simulink model "Electrical_System_2018b_obfs"  (R2019b)
settings: Solver=VariableStepAuto  StartTime=0.0  StopTime=5  RelTol=1e-3  AbsTol=1e-3  EnableMultiTasking=on
InitFcn:
  | Steady_State_Initialisation;
StopFcn:
  | %sscexplore(simlog);
  | %Logging
undefined symbols (not defined in the file): abrlhklxvp, aexgmhuedq, afmfmjnutg, afpphrjpnc, ahuxbyvruc, alarvljztt, amxnyqmnuw, aodrlwvqie, aolhmuplyq, aqpmguuqkg, auesgwirzl, aurophlnng, awamelrhru, ayfhvxflxn, azxkacuhqc, babszerikg, bawhdqanwq, bevoqecvei, bltjvqbchx, bmqsuewujl, bsmyqjfgnf, btvjbsmnve, bywgxqeadw, bziaduxaer, bzmcmdqocb, bzsvyvetat, ccsjnrbsih, cdvenygxwh, cedkrnslhx, cjheorclzs, cjrdshrtqx, ckhavyhcza, ckxewznhlz, cmrcgyiplk, conenicnws, cqkejbgjnn, csfnuwymhe, cunupkhwbh, cwzfvzuxxh, dcadmadufn, dcfponivnv, ddtrqjrhjn, dfhoxvkqas, dfrhtcwpne, dfvomcagjv, djijwylxea, dnmeqksrrm, dnzewbdkaa, dsqcykyxav, dtswwlttmm, ecumpidjtv, edegaywrct, ejjjsmnejc, eknqnehjdz, emvdetzouf, esxbqkbahr, etnkkbreiq, eunoiiiirw, ewewcuedir, fatkfxdhtc ... (+386)
libraries: fl_lib x802, ee_lib x362, fl_ps_legacy_lib x160, nesl_utility x85
(part 13 of 26)

== system Electrical_System_2018b_obfs/Redacted_1221/Redacted_7996/Redacted_1/Redacted_4377/Redacted_6082/Redacted_7871 ==
  Redacted_1150 : ee_lib/Passive/Thermal/Thermal Resistor  R=wnyhcrensu K/W  T_specify=off  T_priority=None  T=hfmwboisgl K  T_nominal_specify=off  T_nominal_unit=K  T_nominal_value=omfgbcxeiw  Q_specify=off  Q_priority=None  Q=jyeccfnuuv W  Q_nominal_specify=off  Q_nominal_unit=W  Q_nominal_value=kbomgljmud
      settings: SourceProductName=Simscape Electrical  SourceProductBaseCode=PS  InternalSimscapePortConfiguration="{\"Bottom\":[],\"Left\":[{\"id\":\"A\",\"label\":\"A\",\"type\":\"foundation.thermal.thermal\"}],\"Right\":[{\"id\":\"B\",\"label\":\"B\",\"type\":\"foundation.thermal.thermal\"}],\"Top\":[]}"
  Redacted_163 : fl_lib/Electrical/Electrical Elements/Switch  R_closed=wdukvpamow Ohm  G_open=xulqxrrjnv 1/Ohm  Threshold=qhmovogayg  i_specify=off  i_priority=None  i=uohgsyxugo A  i_nominal_specify=off  i_nominal_unit=A  i_nominal_value=woebaudwry  v_specify=off  v_priority=None  v=vemtymvmmi V  v_nominal_specify=off  v_nominal_unit=V  v_nominal_value=emvbxsbdsz
      settings: SourceProductName=Simscape
  Redacted_4906 : ee_lib/Semiconductors & Converters/Diode  ModelType=lisxnbujfq  Vf=xetfnwixtl V  Ron=kgggytotak Ohm  Goff=dicegnkmns S  prmExp=fsccnkszzi  I12=rkhncbyaxg A  V12=amfquhqfri V  IS=exemtgyddq A  ec=usfpzulpqi  I1=ugfovaezax A  V1=oljxivlmqp V  RS=dazrmfhoxo Ohm  Tmeas=baitckeesm degC  N_series=hfppshhhyr  N_parallel=rjxplrcndp  Rz=fabwipzqjc Ohm  BV=wyrpdjzqjf V  C_param=qgwqtktiiq  CJ=wbrnhtezpt pF  CJ0=phxqhonqpj pF  VJ=eteydoyhly V  Mgrad=glhtwvcvqy  Vvec=hwlxeyydpv V  Cvec=hxporvcfni pF  FC=gjviwqnvyt  Q_param=ncmzgihjzz  iRM=yvoogxejtg A  iF=qnmfqdbeto A  didt=agfovrodto A/us  trr_factor=frcqxuvvia  trr=hbqrwrvnxm ns  Qrr=fdoqfarsjb s*uA  TT=slfzkacqdx ns  tau=alaeanzbod ns  T_param=nuitneutsg  IS_T2=craloeoioz A  I1_T2=wjjsiamplw A  V1_T2=tewsfpvrmq V  Tmeas2=gxtdnafxpo degC  EG_param=wlioyiusag  EG=cpoejbuzyv eV  XTI_param=dddqpnqtzc  XTI=qrfykfwguz  dBVdT=ucurhhzfza V/K  Tdevice=rczcbfyedr degC  i_specify=off  i_priority=None  i=zzdxemwvng A  i_nominal_specify=off  i_nominal_unit=A  i_nominal_value=kfkirmacjn  v_specify=off  v_priority=None  v=uajyhxnboc V  v_nominal_specify=off  v_nominal_unit=V  v_nominal_value=jqepkydgfh  i_capacitor_specify=off  i_capacitor_priority=None  i_capacitor=rrmwbvgmcc A  i_capacitor_nominal_specify=off  i_capacitor_nominal_unit=A  i_capacitor_nominal_value=pjbytllgoo  v_capacitor_specify=off  v_capacitor_priority=None  v_capacitor=pfzlffxyis V  v_capacitor_nominal_specify=off  v_capacitor_nominal_unit=V  v_capacitor_nominal_value=rwblhtqxum  power_dissipated_specify=off  power_dissipated_priority=None  power_dissipated=ezbuvvjzbd W  power_dissipated_nominal_specify=off  power_dissipated_nominal_unit=W  power_dissipated_nominal_value=bhaqvsgfxr  thermal_network_parameterization=kyfbufrfys  Rth=rdswkjtiwa K/W  Rth_Foster=qshnyhfbmq K/W  thermal_mass_parameterization=gvhwjtzboo  thermal_mass=bdoomqzqok J/K  thermal_mass_Foster=anntstrfod J/K  thermal_time_constant=jfrqkttoqa s  thermal_time_constant_Foster=gslnrdmbpc s  thermal_mass_initial_temperatures=ucxtllsqhb degC
      settings: SourceProductName=Simscape Electrical  InternalSimscapePortConfiguration="{\"Bottom\":[],\"Left\":[{\"id\":\"p\",\"label\":\"\",\"type\":\"foundation.electrical.electrical\"},{\"id\":\"H\",\"label\":\"H\",\"type\":\"foundation.thermal.thermal\"}],\"Right\":[{\"id\":\"n\",\"label\":\"\",\"type\":\"foundation.electrical.electrical\"}],\"Top\":[]}"
  Redacted_5585 : fl_lib/Electrical/Electrical Elements/Switch  R_closed=gnrmopaexe Ohm  G_open=orsehmpisd 1/Ohm  Threshold=uztftemjgo  i_specify=off  i_priority=None  i=beydlfyovg A  i_nominal_specify=off  i_nominal_unit=A  i_nominal_value=iaidkfrlwq  v_specify=off  v_priority=None  v=zwfzhspjsy V  v_nominal_specify=off  v_nominal_unit=V  v_nominal_value=hnducacwcv
      settings: SourceProductName=Simscape
  Redacted_6192 : ee_lib/Semiconductors & Converters/Diode  ModelType=ptnynyqzgs  Vf=tkcshdmnfy V  Ron=etdxecgxkr Ohm  Goff=updvlgzhxi S  prmExp=bdmrzzzqpe  I12=sdcvfvczxq A  V12=qxwxvafkrp V  IS=fjehcmaddz A  ec=rcfxzuuzkz  I1=bbqivzbpbn A  V1=jbzephfaei V  RS=jfqjrslbtb Ohm  Tmeas=nmsknhwbdm degC  N_series=upbnprrhsm  N_parallel=gychkiuesj  Rz=ekjrkafpjm Ohm  BV=izllxqqtbw V  C_param=chrhwjdcia  CJ=zewhvymjzh pF  CJ0=xysumvzksz pF  VJ=plgvwexltq V  Mgrad=lfxmdopixh  Vvec=rhhplxfzfv V  Cvec=btxmrjnrpv pF  FC=gllfdejxcp  Q_param=jqpclwrtup  iRM=uzrdiaqfpb A  iF=zfvqwesedg A  didt=zxsbiuiqyg A/us  trr_factor=sbxmtvfbhj  trr=wpldszobql ns  Qrr=rgofeflbzu s*uA  TT=rydmpcnssa ns  tau=bhbpgrjiqy ns  T_param=utvpupdfuz  IS_T2=hbepvkcqcu A  I1_T2=gjnwhuwyhq A  V1_T2=iliyqurzbt V  Tmeas2=zejnxlzety degC  EG_param=cuajkktsgm  EG=goqdzkjwzg eV  XTI_param=pnvmcekqru  XTI=bkscbkgzda  dBVdT=mkrrrntnlw V/K  Tdevice=tkgdybdqcd degC  i_specify=off  i_priority=None  i=wgjngnbzpn A  i_nominal_specify=off  i_nominal_unit=A  i_nominal_value=ileaslxatl  v_specify=off  v_priority=None  v=agtzcmtlle V  v_nominal_specify=off  v_nominal_unit=V  v_nominal_value=vwqtyzlgqu  i_capacitor_specify=off  i_capacitor_priority=None  i_capacitor=eizgtbmzgc A  i_capacitor_nominal_specify=off  i_capacitor_nominal_unit=A  i_capacitor_nominal_value=vlhejuzknm  v_capacitor_specify=off  v_capacitor_priority=None  v_capacitor=sfnrfbvwbg V  v_capacitor_nominal_specify=off  v_capacitor_nominal_unit=V  v_capacitor_nominal_value=mnvorbtega  power_dissipated_specify=off  power_dissipated_priority=None  power_dissipated=terqltrajz W  power_dissipated_nominal_specify=off  power_dissipated_nominal_unit=W  power_dissipated_nominal_value=akhswoieim  thermal_network_parameterization=aqtnipjlzq  Rth=fvgepqsrwq K/W  Rth_Foster=wcabkcdyac K/W  thermal_mass_parameterization=baajrlnryr  thermal_mass=jkrfnomsau J/K  thermal_mass_Foster=bqnvprbfcb J/K  thermal_time_constant=mwpyhcvjxq s  thermal_time_constant_Foster=nxhccxykrw s  thermal_mass_initial_temperatures=dnnydknyte degC
      settings: SourceProductName=Simscape Electrical  InternalSimscapePortConfiguration="{\"Bottom\":[],\"Left\":[{\"id\":\"p\",\"label\":\"\",\"type\":\"foundation.electrical.electrical\"},{\"id\":\"H\",\"label\":\"H\",\"type\":\"foundation.thermal.thermal\"}],\"Right\":[{\"id\":\"n\",\"label\":\"\",\"type\":\"foundation.electrical.electrical\"}],\"Top\":[]}"
  Redacted_8694 : ee_lib/Passive/Thermal/Thermal Resistor  R=tvtoespfwy K/W  T_specify=off  T_priority=None  T=vzxlafqipt K  T_nominal_specify=off  T_nominal_unit=K  T_nominal_value=cbqqygtnvn  Q_specify=off  Q_priority=None  Q=szwiasewfs W  Q_nominal_specify=off  Q_nominal_unit=W  Q_nominal_value=bbrfndpujl
      settings: SourceProductName=Simscape Electrical  SourceProductBaseCode=PS  InternalSimscapePortConfiguration="{\"Bottom\":[],\"Left\":[{\"id\":\"A\",\"label\":\"A\",\"type\":\"foundation.thermal.thermal\"}],\"Right\":[{\"id\":\"B\",\"label\":\"B\",\"type\":\"foundation.thermal.thermal\"}],\"Top\":[]}"
  Redacted_9167 : ee_lib/Passive/Thermal/Thermal Resistor  R=cjrdshrtqx K/W  T_specify=off  T_priority=None  T=xdavxkvlqw K  T_nominal_specify=off  T_nominal_unit=K  T_nominal_value=bgekadzhxq  Q_specify=off  Q_priority=None  Q=jtdqtarogq W  Q_nominal_specify=off  Q_nominal_unit=W  Q_nominal_value=pabocztlon
      settings: SourceProductName=Simscape Electrical  SourceProductBaseCode=PS  InternalSimscapePortConfiguration="{\"Bottom\":[],\"Left\":[{\"id\":\"A\",\"label\":\"A\",\"type\":\"foundation.thermal.thermal\"}],\"Right\":[{\"id\":\"B\",\"label\":\"B\",\"type\":\"foundation.thermal.thermal\"}],\"Top\":[]}"
  Redacted_2241 : PMIOPort  Side=Left
  Redacted_3211 : PMIOPort  Port=2  Side=Left
  Redacted_9222 : PMIOPort  Port=3  Side=Right
  Redacted_2161 : PMIOPort  Port=4  Side=Right
  Redacted_7477 : PMIOPort  Port=5  Side=Left
  Redacted_8994 : PMIOPort  Port=6  Side=Right
  connections:
  Redacted_6192/LConn1 -- Redacted_3211/RConn1
  Redacted_6192/RConn1 -- Redacted_163/LConn1
  Redacted_4906/LConn2 -- Redacted_9167/LConn1
  Redacted_9222/RConn1 -- Redacted_5585/RConn2
  Redacted_4906/LConn1 -- Redacted_5585/LConn1
  Redacted_2241/RConn1 -- Redacted_4906/RConn1
  Redacted_8694/RConn1 -- Redacted_1150/LConn1 -- Redacted_9167/RConn1
  Redacted_8994/RConn1 -- Redacted_163/RConn1 -- Redacted_5585/RConn1
  Redacted_2161/RConn1 -- Redacted_163/RConn2
  Redacted_1150/RConn1 -- Redacted_7477/RConn1
  Redacted_6192/LConn2 -- Redacted_8694/LConn1

== system Electrical_System_2018b_obfs/Redacted_1221/Redacted_7996/Redacted_1/Redacted_4377/Redacted_6082/Redacted_7884 ==
  Neutral_Negative : Subsystem  VariantControl=Variant1
  Positive_Neutral : Subsystem  VariantControl=Variant3
  Redacted_81 : Subsystem  VariantControl=Variant2
  Redacted_6224 : PMIOPort  Side=Left
  Redacted_4321 : PMIOPort  Port=2  Side=Left
  Redacted_2243 : PMIOPort  Port=3  Side=Left
  Redacted_707 : PMIOPort  Port=4  Side=Right
  Redacted_8636 : PMIOPort  Port=5  Side=Right

== system Electrical_System_2018b_obfs/Redacted_1221/Redacted_7996/Redacted_1/Redacted_4377/Redacted_6082/Redacted_8502 ==
  Neutral_Negative : Subsystem  VariantControl=Variant1
  Positive_Neutral : Subsystem  VariantControl=Variant3
  Redacted_4068 : Subsystem  VariantControl=Variant2
  Redacted_389 : PMIOPort  Side=Left
  Redacted_6488 : PMIOPort  Port=2  Side=Left
  Redacted_5156 : PMIOPort  Port=3  Side=Left
  Redacted_180 : PMIOPort  Port=4  Side=Right
  Redacted_7018 : PMIOPort  Port=5  Side=Right

== system Electrical_System_2018b_obfs/Redacted_1221/Redacted_7996/Redacted_1/Redacted_4377/Redacted_6082/Redacted_8947 ==
  Redacted_1200 : ee_lib/Passive/Thermal/Thermal Resistor  R=conenicnws K/W  T_specify=off  T_priority=None  T=oyfpuqunvc K  T_nominal_specify=off  T_nominal_unit=K  T_nominal_value=hhmaigtkrw  Q_specify=off  Q_priority=None  Q=gvvbtjxjsp W  Q_nominal_specify=off  Q_nominal_unit=W  Q_nominal_value=ytgrxcaawf
      settings: SourceProductName=Simscape Electrical  SourceProductBaseCode=PS  InternalSimscapePortConfiguration="{\"Bottom\":[],\"Left\":[{\"id\":\"A\",\"label\":\"A\",\"type\":\"foundation.thermal.thermal\"}],\"Right\":[{\"id\":\"B\",\"label\":\"B\",\"type\":\"foundation.thermal.thermal\"}],\"Top\":[]}"
  Redacted_2776 : ee_lib/Passive/Thermal/Thermal Resistor  R=xfrdsgmimj K/W  T_specify=off  T_priority=None  T=jqdoourybo K  T_nominal_specify=off  T_nominal_unit=K  T_nominal_value=kshojiwpgf  Q_specify=off  Q_priority=None  Q=hdknkxprge W  Q_nominal_specify=off  Q_nominal_unit=W  Q_nominal_value=lggxgfapwg
      settings: SourceProductName=Simscape Electrical  SourceProductBaseCode=PS  InternalSimscapePortConfiguration="{\"Bottom\":[],\"Left\":[{\"id\":\"A\",\"label\":\"A\",\"type\":\"foundation.thermal.thermal\"}],\"Right\":[{\"id\":\"B\",\"label\":\"B\",\"type\":\"foundation.thermal.thermal\"}],\"Top\":[]}"
  Redacted_3753 : fl_lib/Electrical/Electrical Elements/Switch  R_closed=myhzxdbcyd Ohm  G_open=tgukgpdyma 1/Ohm  Threshold=rhadczetof  i_specify=off  i_priority=None  i=tlxbnxojhu A  i_nominal_specify=off  i_nominal_unit=A  i_nominal_value=oqbnzgqfjp  v_specify=off  v_priority=None  v=nhvfxaeqlj V  v_nominal_specify=off  v_nominal_unit=V  v_nominal_value=xplygqiccy
      settings: SourceProductName=Simscape
  Redacted_4699 : ee_lib/Semiconductors & Converters/Diode  ModelType=okioahdqsa  Vf=biiykosjxn V  Ron=ciffxclmjc Ohm  Goff=fvgtukyouc S  prmExp=xfckdxdmby  I12=frheejtyjl A  V12=gimvccaqda V  IS=wbwdsgcbei A  ec=ekagsdlnjh  I1=mwpudxxhbv A  V1=lmydwavwlr V  RS=ewsjxwtbez Ohm  Tmeas=qktzrtaqmp degC  N_series=vmryfhrwop  N_parallel=mjdqxbceby  Rz=mcmzhynykr Ohm  BV=lsdxbqfxay V  C_param=bbriskmjxm  CJ=embugfvnon pF  CJ0=lisphtthyv pF  VJ=kektwkntmb V  Mgrad=kmnuxclqxb  Vvec=ubnzixryip V  Cvec=wodzzuhisg pF  FC=oslwfyuxap  Q_param=snjyccpyvs  iRM=rbqvugpaid A  iF=vkiwaflpcp A  didt=piepoonbzm A/us  trr_factor=uinijxvxfw  trr=zcafmrqrge ns  Qrr=rpzpcfdhhu s*uA  TT=tiqvphdbkk ns  tau=umrnemkplk ns  T_param=qrurbakqcm  IS_T2=xdewdelbdy A  I1_T2=gquvzxlvxd A  V1_T2=pdpxwcqlqf V  Tmeas2=wjworhtoap degC  EG_param=labsejfvmg  EG=ttgxidatuc eV  XTI_param=ojrnxozkll  XTI=rozlwnnkry  dBVdT=pccpuhnmah V/K  Tdevice=tuzidgepzf degC  i_specify=off  i_priority=None  i=qbnehebxse A  i_nominal_specify=off  i_nominal_unit=A  i_nominal_value=mibocxegog  v_specify=off  v_priority=None  v=kqsuidjkks V  v_nominal_specify=off  v_nominal_unit=V  v_nominal_value=fbbyhdwpgw  i_capacitor_specify=off  i_capacitor_priority=None  i_capacitor=ajlpnxcugc A  i_capacitor_nominal_specify=off  i_capacitor_nominal_unit=A  i_capacitor_nominal_value=kogaemqmtt  v_capacitor_specify=off  v_capacitor_priority=None  v_capacitor=bhiwsiovzj V  v_capacitor_nominal_specify=off  v_capacitor_nominal_unit=V  v_capacitor_nominal_value=nclaqhshnb  power_dissipated_specify=off  power_dissipated_priority=None  power_dissipated=cptsujrpwk W  power_dissipated_nominal_specify=off  power_dissipated_nominal_unit=W  power_dissipated_nominal_value=edquulnadh  thermal_network_parameterization=pshljmcicg  Rth=pxuolvhflb K/W  Rth_Foster=efhwuoeamy K/W  thermal_mass_parameterization=rqnbetowsy  thermal_mass=pgrizesowt J/K  thermal_mass_Foster=exxnfsiexd J/K  thermal_time_constant=tympttoyhy s  thermal_time_constant_Foster=fdehqpjaek s  thermal_mass_initial_temperatures=bvqvmotyla degC
      settings: SourceProductName=Simscape Electrical  InternalSimscapePortConfiguration="{\"Bottom\":[],\"Left\":[{\"id\":\"p\",\"label\":\"\",\"type\":\"foundation.electrical.electrical\"},{\"id\":\"H\",\"label\":\"H\",\"type\":\"foundation.thermal.thermal\"}],\"Right\":[{\"id\":\"n\",\"label\":\"\",\"type\":\"foundation.electrical.electrical\"}],\"Top\":[]}"
  Redacted_6350 : ee_lib/Passive/Thermal/Thermal Resistor  R=yrxhjsyicv K/W  T_specify=off  T_priority=None  T=mkgjpjryvb K  T_nominal_specify=off  T_nominal_unit=K  T_nominal_value=rimnnrkxgy  Q_specify=off  Q_priority=None  Q=moghwbombz W  Q_nominal_specify=off  Q_nominal_unit=W  Q_nominal_value=ltiqiabezd
      settings: SourceProductName=Simscape Electrical  SourceProductBaseCode=PS  InternalSimscapePortConfiguration="{\"Bottom\":[],\"Left\":[{\"id\":\"A\",\"label\":\"A\",\"type\":\"foundation.thermal.thermal\"}],\"Right\":[{\"id\":\"B\",\"label\":\"B\",\"type\":\"foundation.thermal.thermal\"}],\"Top\":[]}"
  Redacted_7029 : fl_lib/Electrical/Electrical Elements/Switch  R_closed=myhcjbwtor Ohm  G_open=xbozcrpyih 1/Ohm  Threshold=cunupkhwbh  i_specify=off  i_priority=None  i=prynjnashs A  i_nominal_specify=off  i_nominal_unit=A  i_nominal_value=hagfxzjsld  v_specify=off  v_priority=None  v=aqyrbgibll V  v_nominal_specify=off  v_nominal_unit=V  v_nominal_value=faydptnycf
      settings: SourceProductName=Simscape
  Redacted_7102 : ee_lib/Passive/Thermal/Thermal Resistor  R=nbzdnvocwa K/W  T_specify=off  T_priority=None  T=fmjnhsptuu K  T_nominal_specify=off  T_nominal_unit=K  T_nominal_value=jbgjaqctax  Q_specify=off  Q_priority=None  Q=fwmhforkhj W  Q_nominal_specify=off  Q_nominal_unit=W  Q_nominal_value=ntnzagimnx
      settings: SourceProductName=Simscape Electrical  SourceProductBaseCode=PS  InternalSimscapePortConfiguration="{\"Bottom\":[],\"Left\":[{\"id\":\"A\",\"label\":\"A\",\"type\":\"foundation.thermal.thermal\"}],\"Right\":[{\"id\":\"B\",\"label\":\"B\",\"type\":\"foundation.thermal.thermal\"}],\"Top\":[]}"
  Redacted_7564 : ee_lib/Semiconductors & Converters/Diode  ModelType=nzjlvuoikn  Vf=xcqjsaaovm V  Ron=fkxfatroeg Ohm  Goff=xlystovpxi S  prmExp=jgotoknapp  I12=tfnmviaryi A  V12=jszilbxvdd V  IS=sxnnygsvvh A  ec=prpymivtsf  I1=taqpcdkgmt A  V1=dyhqbqrjzo V  RS=jeqvinzske Ohm  Tmeas=xmdysrekbb degC  N_series=dgxjmifyxk  N_parallel=bdrkhzkiko  Rz=cyzhxvwwxk Ohm  BV=hncdeuwdkt V  C_param=bciflpqhvj  CJ=tattmalnku pF  CJ0=wvdwpbdajw pF  VJ=mrbbsihqag V  Mgrad=byylwbotni  Vvec=cqinlhejdr V  Cvec=xewqpzizht pF  FC=bltnzhtfty  Q_param=qjidjcpzmq  iRM=pmjyefmfqa A  iF=itopnidmku A  didt=bigtioflxe A/us  trr_factor=kvyspqeanm  trr=koacayohkq ns  Qrr=fdpsfuffyd s*uA  TT=zsxzrazayp ns  tau=kykdroosyj ns  T_param=vbclpvccfu  IS_T2=funngziywg A  I1_T2=wicrbycbdq A  V1_T2=vgdrxhmjnf V  Tmeas2=eollgrgwfz degC  EG_param=wzkpxvlami  EG=gnmutqrkjg eV  XTI_param=crjuukcasz  XTI=ymywhallih  dBVdT=zjptrtddls V/K  Tdevice=gnfncpylll degC  i_specify=off  i_priority=None  i=fecvdzvdqq A  i_nominal_specify=off  i_nominal_unit=A  i_nominal_value=vtwsncvxqu  v_specify=off  v_priority=None  v=fuemubwutc V  v_nominal_specify=off  v_nominal_unit=V  v_nominal_value=ohpskerenl  i_capacitor_specify=off  i_capacitor_priority=None  i_capacitor=fjydyicunb A  i_capacitor_nominal_specify=off  i_capacitor_nominal_unit=A  i_capacitor_nominal_value=prrwxpzods  v_capacitor_specify=off  v_capacitor_priority=None  v_capacitor=xsnisfvufl V  v_capacitor_nominal_specify=off  v_capacitor_nominal_unit=V  v_capacitor_nominal_value=roccqlotwg  power_dissipated_specify=off  power_dissipated_priority=None  power_dissipated=xfylhqvksm W  power_dissipated_nominal_specify=off  power_dissipated_nominal_unit=W  power_dissipated_nominal_value=pgypdqdrjk  thermal_network_parameterization=hzusrmlwsx  Rth=brajdypygx K/W  Rth_Foster=cgyaeferoq K/W  thermal_mass_parameterization=czoqewtctg  thermal_mass=xchjhblwgw J/K  thermal_mass_Foster=lstamqxuph J/K  thermal_time_constant=vqnjlbkxab s  thermal_time_constant_Foster=lrckilnlvz s  thermal_mass_initial_temperatures=qgcdwjydqd degC
      settings: SourceProductName=Simscape Electrical  InternalSimscapePortConfiguration="{\"Bottom\":[],\"Left\":[{\"id\":\"p\",\"label\":\"\",\"type\":\"foundation.electrical.electrical\"},{\"id\":\"H\",\"label\":\"H\",\"type\":\"foundation.thermal.thermal\"}],\"Right\":[{\"id\":\"n\",\"label\":\"\",\"type\":\"foundation.electrical.electrical\"}],\"Top\":[]}"
  Redacted_7588 : ee_lib/Semiconductors & Converters/Diode  ModelType=odluhstpuq  Vf=okyirdnfjx V  Ron=mapmrrrdjd Ohm  Goff=bviukcoyfs S  prmExp=vclubligzd  I12=svcnamrwpx A  V12=cfavrzhwjm V  IS=ndjntmrdax A  ec=jybmppblnf  I1=xwbzkojill A  V1=uhudrubuie V  RS=ouaxzubtjl Ohm  Tmeas=ajhpuloixi degC  N_series=shgcbsfbub  N_parallel=mkqgqoyeam  Rz=hvnrlffdia Ohm  BV=pzbqztfsns V  C_param=lavqdifgpp  CJ=gljxgypfmd pF  CJ0=oabrsrprvz pF  VJ=bhnkzaolxf V  Mgrad=cnntipdjdo  Vvec=umbplbvvci V  Cvec=uyrzvfnogt pF  FC=xfstmxzgmk  Q_param=ikdwbmwcpm  iRM=dfocryvzhl A  iF=fufpnqgtwg A  didt=dzifmwnrtb A/us  trr_factor=jwtwxmuuxw  trr=pkchaoncoz ns  Qrr=pvdwdaonye s*uA  TT=tdxxlpvijc ns  tau=zqckzcange ns  T_param=aivfrewmny  IS_T2=lyqtiaxegv A  I1_T2=qpjbnvocgz A  V1_T2=vkfdtsaqjr V  Tmeas2=upqktjuvjp degC  EG_param=zrarctnbos  EG=jqgbqmxvws eV  XTI_param=lxwpfrhxyo  XTI=smupagfiul  dBVdT=qhdgxbkeme V/K  Tdevice=afxxhsnjeq degC  i_specify=off  i_priority=None  i=zfsllfgnmn A  i_nominal_specify=off  i_nominal_unit=A  i_nominal_value=tfhurexabo  v_specify=off  v_priority=None  v=juhufvbmad V  v_nominal_specify=off  v_nominal_unit=V  v_nominal_value=ovmdqfbmpz  i_capacitor_specify=off  i_capacitor_priority=None  i_capacitor=cpkalirwmj A  i_capacitor_nominal_specify=off  i_capacitor_nominal_unit=A  i_capacitor_nominal_value=cukofimbps  v_capacitor_specify=off  v_capacitor_priority=None  v_capacitor=svzxprpfnc V  v_capacitor_nominal_specify=off  v_capacitor_nominal_unit=V  v_capacitor_nominal_value=efigblkcuc  power_dissipated_specify=off  power_dissipated_priority=None  power_dissipated=nbxvqpojmg W  power_dissipated_nominal_specify=off  power_dissipated_nominal_unit=W  power_dissipated_nominal_value=qazgeznxoo  thermal_network_parameterization=mawvfhuqlc  Rth=aorgfikkxj K/W  Rth_Foster=yidglncciz K/W  thermal_mass_parameterization=mbkqhjofgx  thermal_mass=tdcnydwamw J/K  thermal_mass_Foster=ymwvmeergr J/K  thermal_time_constant=mrvxjciynj s  thermal_time_constant_Foster=pduwmiqqfq s  thermal_mass_initial_temperatures=xyvzcgqxko degC
      settings: SourceProductName=Simscape Electrical  InternalSimscapePortConfiguration="{\"Bottom\":[],\"Left\":[{\"id\":\"p\",\"label\":\"\",\"type\":\"foundation.electrical.electrical\"},{\"id\":\"H\",\"label\":\"H\",\"type\":\"foundation.thermal.thermal\"}],\"Right\":[{\"id\":\"n\",\"label\":\"\",\"type\":\"foundation.electrical.electrical\"}],\"Top\":[]}"
  Redacted_7943 : ee_lib/Semiconductors & Converters/Diode  ModelType=huwnyzhagg  Vf=uhdwajzbci V  Ron=umdafdpiie Ohm  Goff=wflpqropjk S  prmExp=snfjdxnypd  I12=llhdfxbhig A  V12=pdmhgeajec V  IS=nhbhwhdpog A  ec=tkilreksdk  I1=bgwngczvyl A  V1=wixmbbwapc V  RS=qcsovublns Ohm  Tmeas=bqbiajtrmn degC  N_series=twrzdtxsxs  N_parallel=yamvajjsau  Rz=onmncvbjbt Ohm  BV=zdnzokfxlk V  C_param=qthgugszua  CJ=kmuxknphwi pF  CJ0=vsucecbflq pF  VJ=fycxbfoksn V  Mgrad=xkpjcofnjn  Vvec=ojzdvhtmbe V  Cvec=bscefekwwt pF  FC=jrtwuwdita  Q_param=cepjqanuzl  iRM=auifzbaagq A  iF=ggvxvxeroq A  didt=upduwbdmhl A/us  trr_factor=iwbpdhvywt  trr=yhdbydzbts ns  Qrr=fscdweiuof s*uA  TT=snshdcawru ns  tau=wajkwtjuth ns  T_param=auvvsbsdpl  IS_T2=bstuzffxgu A  I1_T2=jmvsfyaobh A  V1_T2=rkzggaqmmy V  Tmeas2=kkjgyfusfv degC  EG_param=aaodjuuynt  EG=qhmkilzbox eV  XTI_param=vqwxmrtbso  XTI=xgaemwxaak  dBVdT=iqehuznwgn V/K  Tdevice=cldkwcsoqu degC  i_specify=off  i_priority=None  i=idcyovpjxl A  i_nominal_specify=off  i_nominal_unit=A  i_nominal_value=pxuqftausp  v_specify=off  v_priority=None  v=latjtqsste V  v_nominal_specify=off  v_nominal_unit=V  v_nominal_value=vlfbwzysbm  i_capacitor_specify=off  i_capacitor_priority=None  i_capacitor=fxbytskqnk A  i_capacitor_nominal_specify=off  i_capacitor_nominal_unit=A  i_capacitor_nominal_value=qswqedwltm  v_capacitor_specify=off  v_capacitor_priority=None  v_capacitor=nnywysrwxl V  v_capacitor_nominal_specify=off  v_capacitor_nominal_unit=V  v_capacitor_nominal_value=kcesdbxuoj  power_dissipated_specify=off  power_dissipated_priority=None  power_dissipated=rjeaxrgaob W  power_dissipated_nominal_specify=off  power_dissipated_nominal_unit=W  power_dissipated_nominal_value=tpzvmpkopo  thermal_network_parameterization=tpzgtvxnfw  Rth=dlctzipjor K/W  Rth_Foster=omutbgrari K/W  thermal_mass_parameterization=zsuosqjyzh  thermal_mass=agpurubbbx J/K  thermal_mass_Foster=gojuilhson J/K  thermal_time_constant=blcffyxhgw s  thermal_time_constant_Foster=bvfynyveyr s  thermal_mass_initial_temperatures=oqnejpxvbw degC
      settings: SourceProductName=Simscape Electrical  InternalSimscapePortConfiguration="{\"Bottom\":[],\"Left\":[{\"id\":\"p\",\"label\":\"\",\"type\":\"foundation.electrical.electrical\"},{\"id\":\"H\",\"label\":\"H\",\"type\":\"foundation.thermal.thermal\"}],\"Right\":[{\"id\":\"n\",\"label\":\"\",\"type\":\"foundation.electrical.electrical\"}],\"Top\":[]}"
  Redacted_8651 : ee_lib/Semiconductors & Converters/Diode  ModelType=skgooupexc  Vf=boumedklyp V  Ron=ijvoavmnlu Ohm  Goff=cmdacawmhi S  prmExp=dylqcjyybj  I12=rhpkdiqtuc A  V12=ckmlhkotyk V  IS=jnpojtuxdv A  ec=ecqncdbiea  I1=xlctmcvyei A  V1=duzuttqxti V  RS=cnpprwofhs Ohm  Tmeas=sauusbcwcf degC  N_series=xaitwekewt  N_parallel=tpxpxznjnf  Rz=wjyvnwlafu Ohm  BV=wiyvqwbloq V  C_param=zqduolbfwx  CJ=hpgdqwckxb pF  CJ0=azvouvolma pF  VJ=jkfcgwafsp V  Mgrad=fwzxrlkoob  Vvec=obtficftkq V  Cvec=yvdztdtopd pF  FC=dsnbkwwfpf  Q_param=yvvpfaokvu  iRM=wmoupborte A  iF=grzjolhdzl A  didt=zeuybymzvb A/us  trr_factor=xgvcrwgnha  trr=xcvmkapoku ns  Qrr=xdhpfspren s*uA  TT=zdnzbhmtkp ns  tau=gbkrfessaz ns  T_param=aorxxxflrb  IS_T2=yhbakacbpw A  I1_T2=tkkccpjvrs A  V1_T2=tyvkrwsznz V  Tmeas2=zsfnhormbn degC  EG_param=llsagzfltn  EG=vymtdamjzw eV  XTI_param=cjfetnxdvu  XTI=ifdjojcxmh  dBVdT=yrzrjlpemk V/K  Tdevice=hynxjwzdho degC  i_specify=off  i_priority=None  i=lckcddvpcc A  i_nominal_specify=off  i_nominal_unit=A  i_nominal_value=yiqaeiaxxn  v_specify=off  v_priority=None  v=iycopiwoye V  v_nominal_specify=off  v_nominal_unit=V  v_nominal_value=qvhznolemy  i_capacitor_specify=off  i_capacitor_priority=None  i_capacitor=zkinjigaml A  i_capacitor_nominal_specify=off  i_capacitor_nominal_unit=A  i_capacitor_nominal_value=objhxdwknb  v_capacitor_specify=off  v_capacitor_priority=None  v_capacitor=ugvbmprvdv V  v_capacitor_nominal_specify=off  v_capacitor_nominal_unit=V  v_capacitor_nominal_value=pqcoklrxbg  power_dissipated_specify=off  power_dissipated_priority=None  power_dissipated=dyovkxndty W  power_dissipated_nominal_specify=off  power_dissipated_nominal_unit=W  power_dissipated_nominal_value=lkqnimcieb  thermal_network_parameterization=fkczmhiwkd  Rth=pgkcebyssc K/W  Rth_Foster=vvqbxikvgn K/W  thermal_mass_parameterization=eztvlfptdb  thermal_mass=gihuphwqhu J/K  thermal_mass_Foster=dfshmowzki J/K  thermal_time_constant=qkhynikdrk s  thermal_time_constant_Foster=fsnuafgxeg s  thermal_mass_initial_temperatures=cptnoispoo degC
      settings: SourceProductName=Simscape Electrical  InternalSimscapePortConfiguration="{\"Bottom\":[],\"Left\":[{\"id\":\"p\",\"label\":\"\",\"type\":\"foundation.electrical.electrical\"},{\"id\":\"H\",\"label\":\"H\",\"type\":\"foundation.thermal.thermal\"}],\"Right\":[{\"id\":\"n\",\"label\":\"\",\"type\":\"foundation.electrical.electrical\"}],\"Top\":[]}"
  Redacted_9946 : fl_lib/Electrical/Electrical Elements/Switch  R_closed=fueibbmuph Ohm  G_open=whmrzixjuv 1/Ohm  Threshold=abrlhklxvp  i_specify=off  i_priority=None  i=bgqhsybdvn A  i_nominal_specify=off  i_nominal_unit=A  i_nominal_value=avqltruyiy  v_specify=off  v_priority=None  v=cyldwpxbuh V  v_nominal_specify=off  v_nominal_unit=V  v_nominal_value=mjhmtfemhi
      settings: SourceProductName=Simscape
  Redacted_1580 : PMIOPort  Side=Left
  Redacted_5022 : PMIOPort  Port=2  Side=Left
  Redacted_2222 : PMIOPort  Port=3  Side=Left
  Redacted_3136 : PMIOPort  Port=4  Side=Right
  Redacted_6675 : PMIOPort  Port=5  Side=Right
  Redacted_8346 : PMIOPort  Port=6  Side=Right
  Redacted_105 : PMIOPort  Port=7  Side=Left
  Redacted_2281 : PMIOPort  Port=8  Side=Right
  connections:
  Redacted_8651/LConn2 -- Redacted_6350/LConn1
  Redacted_7102/RConn1 -- Redacted_105/RConn1
  Redacted_7943/LConn2 -- Redacted_2776/LConn1 -- Redacted_4699/LConn2
  Redacted_7943/RConn1 -- Redacted_3753/LConn1 -- Redacted_4699/LConn1
  Redacted_6675/RConn1 -- Redacted_9946/RConn2
  Redacted_7029/RConn1 -- Redacted_9946/RConn1 -- Redacted_3753/RConn1 -- Redacted_2281/RConn1
  Redacted_8346/RConn1 -- Redacted_3753/RConn2
  Redacted_4699/RConn1 -- Redacted_2222/RConn1 -- Redacted_7943/LConn1
  Redacted_1200/RConn1 -- Redacted_7102/LConn1 -- Redacted_2776/RConn1 -- Redacted_6350/RConn1
  Redacted_7588/RConn1 -- Redacted_1580/RConn1 -- Redacted_7564/LConn1
  Redacted_7564/RConn1 -- Redacted_7029/LConn1 -- Redacted_7588/LConn1
  Redacted_3136/RConn1 -- Redacted_7029/RConn2
  Redacted_7588/LConn2 -- Redacted_7564/LConn2 -- Redacted_1200/LConn1
  Redacted_8651/RConn1 -- Redacted_9946/LConn1
  Redacted_8651/LConn1 -- Redacted_5022/RConn1

== system Electrical_System_2018b_obfs/Redacted_1221/Redacted_7996/Redacted_1/Redacted_4377/Redacted_6082/Redacted_9034 ==
  Neutral_Negative : Subsystem  VariantControl=Variant1
  Positive_Neutral : Subsystem  VariantControl=Variant3
  Redacted_4182 : Subsystem  VariantControl=Variant2
  Redacted_4887 : PMIOPort  Side=Left
  Redacted_5529 : PMIOPort  Port=2  Side=Left
  Redacted_4069 : PMIOPort  Port=3  Side=Left
  Redacted_1826 : PMIOPort  Port=4  Side=Right
  Redacted_1222 : PMIOPort  Port=5  Side=Right

== system Electrical_System_2018b_obfs/Redacted_1221/Redacted_7996/Redacted_1/Redacted_4377/Redacted_6082/Redacted_9175 ==
  Redacted_190 : fl_lib/Electrical/Electrical Elements/Switch  R_closed=fepusinwsd Ohm  G_open=sjwayaisbu 1/Ohm  Threshold=zizvtnqmmi  i_specify=off  i_priority=None  i=encinxtjft A  i_nominal_specify=off  i_nominal_unit=A  i_nominal_value=gtziqetnpy  v_specify=off  v_priority=None  v=iegjwximjs V  v_nominal_specify=off  v_nominal_unit=V  v_nominal_value=kdesewwsrp
      settings: SourceProductName=Simscape
  Redacted_3040 : ee_lib/Passive/Thermal/Thermal Resistor  R=obfkrrtkcz K/W  T_specify=off  T_priority=None  T=rtkamgxcrd K  T_nominal_specify=off  T_nominal_unit=K  T_nominal_value=bpzfjmxahn  Q_specify=off  Q_priority=None  Q=hqotbiagtp W  Q_nominal_specify=off  Q_nominal_unit=W  Q_nominal_value=ygrtgietmq
      settings: SourceProductName=Simscape Electrical  SourceProductBaseCode=PS  InternalSimscapePortConfiguration="{\"Bottom\":[],\"Left\":[{\"id\":\"A\",\"label\":\"A\",\"type\":\"foundation.thermal.thermal\"}],\"Right\":[{\"id\":\"B\",\"label\":\"B\",\"type\":\"foundation.thermal.thermal\"}],\"Top\":[]}"
  Redacted_4841 : ee_lib/Semiconductors & Converters/Diode  ModelType=rbznrmeoeu  Vf=cohupiidqm V  Ron=fgoazeflfv Ohm  Goff=zhgdntbgyc S  prmExp=sqtnmzyces  I12=ghumtexxod A  V12=ryuivsynyp V  IS=zvtyiafsje A  ec=nbbckqrsca  I1=vvnwgjhbel A  V1=blcwxgugdf V  RS=qcorpcyvcy Ohm  Tmeas=ckjljgosyn degC  N_series=svmyqwlzvl  N_parallel=qyrmvajmsz  Rz=estapunyjj Ohm  BV=farqrpcpvl V  C_param=lrybxatfhg  CJ=uvbqcvgqiy pF  CJ0=lxclnyvvbo pF  VJ=oxjlzamklu V  Mgrad=ytaabhzbob  Vvec=nnmrambevz V  Cvec=wgogoztzrr pF  FC=qrtvwbdqsa  Q_param=iztgtuynho  iRM=clmjvqaesa A  iF=bvkvfnmhiu A  didt=kafxplzqrb A/us  trr_factor=nvnoyeprol  trr=soxptuevfa ns  Qrr=wfejkrfyve s*uA  TT=pywmdvejog ns  tau=bigtovpzkb ns  T_param=pokcfhrpif  IS_T2=ctmxcqrvfi A  I1_T2=wgvikudhch A  V1_T2=urasrwbdwu V  Tmeas2=uprvkustxb degC  EG_param=ihveuboixo  EG=ptejfeznid eV  XTI_param=jhchwrybdp  XTI=sxraamqqfp  dBVdT=rktpslarrn V/K  Tdevice=xxpawatkyi degC  i_specify=off  i_priority=None  i=ujzxybkfga A  i_nominal_specify=off  i_nominal_unit=A  i_nominal_value=xonmzaaonh  v_specify=off  v_priority=None  v=mwvcemnvaa V  v_nominal_specify=off  v_nominal_unit=V  v_nominal_value=kbeepvsgqz  i_capacitor_specify=off  i_capacitor_priority=None  i_capacitor=qxlfjzwxqp A  i_capacitor_nominal_specify=off  i_capacitor_nominal_unit=A  i_capacitor_nominal_value=isnbzzmude  v_capacitor_specify=off  v_capacitor_priority=None  v_capacitor=imyyegylhv V  v_capacitor_nominal_specify=off  v_capacitor_nominal_unit=V  v_capacitor_nominal_value=qnwvvgxfdn  power_dissipated_specify=off  power_dissipated_priority=None  power_dissipated=uhlataobag W  power_dissipated_nominal_specify=off  power_dissipated_nominal_unit=W  power_dissipated_nominal_value=shjjmztoit  thermal_network_parameterization=dnfemugqbf  Rth=tbkhycnsnf K/W  Rth_Foster=reqetgenti K/W  thermal_mass_parameterization=espvpmvftt  thermal_mass=oejnqshmxj J/K  thermal_mass_Foster=ngmehkzaij J/K  thermal_time_constant=cfsdhnktyb s  thermal_time_constant_Foster=oypydrqsyx s  thermal_mass_initial_temperatures=hlnadppage degC
      settings: SourceProductName=Simscape Electrical  InternalSimscapePortConfiguration="{\"Bottom\":[],\"Left\":[{\"id\":\"p\",\"label\":\"\",\"type\":\"foundation.electrical.electrical\"},{\"id\":\"H\",\"label\":\"H\",\"type\":\"foundation.thermal.thermal\"}],\"Right\":[{\"id\":\"n\",\"label\":\"\",\"type\":\"foundation.electrical.electrical\"}],\"Top\":[]}"
  Redacted_6531 : fl_lib/Electrical/Electrical Elements/Switch  R_closed=qrehwkffpu Ohm  G_open=rgvojfvhps 1/Ohm  Threshold=qvwygodojk  i_specify=off  i_priority=None  i=muktgalobr A  i_nominal_specify=off  i_nominal_unit=A  i_nominal_value=htembpubcm  v_specify=off  v_priority=None  v=fbaqrdqffe V  v_nominal_specify=off  v_nominal_unit=V  v_nominal_value=ruvanaztjl
      settings: SourceProductName=Simscape
  Redacted_6791 : ee_lib/Passive/Thermal/Thermal Resistor  R=togppmmsum K/W  T_specify=off  T_priority=None  T=ewewcuedir K  T_nominal_specify=off  T_nominal_unit=K  T_nominal_value=hnigxokuoz  Q_specify=off  Q_priority=None  Q=hwywgkxcwt W  Q_nominal_specify=off  Q_nominal_unit=W  Q_nominal_value=pjojjlvphl
      settings: SourceProductName=Simscape Electrical  SourceProductBaseCode=PS  InternalSimscapePortConfiguration="{\"Bottom\":[],\"Left\":[{\"id\":\"A\",\"label\":\"A\",\"type\":\"foundation.thermal.thermal\"}],\"Right\":[{\"id\":\"B\",\"label\":\"B\",\"type\":\"foundation.thermal.thermal\"}],\"Top\":[]}"
  Redacted_8321 : ee_lib/Semiconductors & Converters/Diode  ModelType=ubybrclmwm  Vf=lciqexaceh V  Ron=ljddmpvkof Ohm  Goff=frccxsuwjg S  prmExp=wuooxypqqf  I12=nhybrofyli A  V12=irwnpdfszl V  IS=sqoylpljvt A  ec=xhcvlpuguu  I1=cnayzqobxj A  V1=qxodfcctdw V  RS=bimvobbxbz Ohm  Tmeas=omhyaidhuy degC  N_series=opsadzyoac  N_parallel=vfuutvansz  Rz=swjewafqtp Ohm  BV=uhqmvahezk V  C_param=armxkgnczf  CJ=xgszpsejne pF  CJ0=fmoixcodat pF  VJ=orzlpgatux V  Mgrad=nodcgjthfp  Vvec=hqqpplwkvd V  Cvec=gmhoaqlwwo pF  FC=ucqjbbzkqf  Q_param=tdlyjvbada  iRM=dzmeggbfwj A  iF=ooynoxqglh A  didt=pizbmqopdr A/us  trr_factor=jwjvjuntbo  trr=ajnustfegb ns  Qrr=ucnrlsxhaw s*uA  TT=xzyydvdnoz ns  tau=ffqrqgxofo ns  T_param=wjdgrbukmw  IS_T2=cmubsfcuiu A  I1_T2=ajxovuxnps A  V1_T2=wbwdzvwxii V  Tmeas2=etnrjarcrm degC  EG_param=rromvawzpl  EG=xlubbarmng eV  XTI_param=sxmvwhlaen  XTI=ubkscpwrxq  dBVdT=gcgrsxrmbr V/K  Tdevice=hicvhwdftj degC  i_specify=off  i_priority=None  i=clqbewupwz A  i_nominal_specify=off  i_nominal_unit=A  i_nominal_value=ojquwrvnup  v_specify=off  v_priority=None  v=qdgeikhcfd V  v_nominal_specify=off  v_nominal_unit=V  v_nominal_value=zmmyqujkfm  i_capacitor_specify=off  i_capacitor_priority=None  i_capacitor=unmufjoxtr A  i_capacitor_nominal_specify=off  i_capacitor_nominal_unit=A  i_capacitor_nominal_value=pjtcifagny  v_capacitor_specify=off  v_capacitor_priority=None  v_capacitor=ienwbakehg V  v_capacitor_nominal_specify=off  v_capacitor_nominal_unit=V  v_capacitor_nominal_value=hyfjwcqjlw  power_dissipated_specify=off  power_dissipated_priority=None  power_dissipated=kamfvdccnw W  power_dissipated_nominal_specify=off  power_dissipated_nominal_unit=W  power_dissipated_nominal_value=ruufiykqfg  thermal_network_parameterization=rxpzlgddeq  Rth=whgdtwbinu K/W  Rth_Foster=aluvftlbib K/W  thermal_mass_parameterization=uhtaedpyom  thermal_mass=wbvtvqluqn J/K  thermal_mass_Foster=becrvvdvrg J/K  thermal_time_constant=arapyicwyx s  thermal_time_constant_Foster=atyjgrmjfj s  thermal_mass_initial_temperatures=iyuewlykif degC
      settings: SourceProductName=Simscape Electrical  InternalSimscapePortConfiguration="{\"Bottom\":[],\"Left\":[{\"id\":\"p\",\"label\":\"\",\"type\":\"foundation.electrical.electrical\"},{\"id\":\"H\",\"label\":\"H\",\"type\":\"foundation.thermal.thermal\"}],\"Right\":[{\"id\":\"n\",\"label\":\"\",\"type\":\"foundation.electrical.electrical\"}],\"Top\":[]}"
  Redacted_8744 : ee_lib/Passive/Thermal/Thermal Resistor  R=pslxtkyais K/W  T_specify=off  T_priority=None  T=xvxbtjagyi K  T_nominal_specify=off  T_nominal_unit=K  T_nominal_value=xhgruaelob  Q_specify=off  Q_priority=None  Q=htzftxlgll W  Q_nominal_specify=off  Q_nominal_unit=W  Q_nominal_value=kkksntoxni
      settings: SourceProductName=Simscape Electrical  SourceProductBaseCode=PS  InternalSimscapePortConfiguration="{\"Bottom\":[],\"Left\":[{\"id\":\"A\",\"label\":\"A\",\"type\":\"foundation.thermal.thermal\"}],\"Right\":[{\"id\":\"B\",\"label\":\"B\",\"type\":\"foundation.thermal.thermal\"}],\"Top\":[]}"
  Redacted_708 : PMIOPort  Side=Left
  Redacted_5765 : PMIOPort  Port=2  Side=Left
  Redacted_5734 : PMIOPort  Port=3  Side=Right
  Redacted_3054 : PMIOPort  Port=4  Side=Right
  Redacted_8091 : PMIOPort  Port=5  Side=Left
  Redacted_9229 : PMIOPort  Port=6  Side=Right
  connections:
  Redacted_8321/LConn2 -- Redacted_8744/LConn1
  Redacted_3040/RConn1 -- Redacted_8091/RConn1
  Redacted_3054/RConn1 -- Redacted_6531/RConn2
  Redacted_190/RConn1 -- Redacted_6531/RConn1 -- Redacted_9229/RConn1
  Redacted_6791/RConn1 -- Redacted_3040/LConn1 -- Redacted_8744/RConn1
  Redacted_708/RConn1 -- Redacted_4841/RConn1
  Redacted_4841/LConn1 -- Redacted_190/LConn1
  Redacted_5734/RConn1 -- Redacted_190/RConn2
  Redacted_4841/LConn2 -- Redacted_6791/LConn1
  Redacted_8321/RConn1 -- Redacted_6531/LConn1
  Redacted_8321/LConn1 -- Redacted_5765/RConn1

== system Electrical_System_2018b_obfs/Redacted_1221/Redacted_7996/Redacted_1/Redacted_4377/Redacted_6082/Redacted_9572 ==
  Neutral_Negative : Subsystem  VariantControl=Variant1
  Positive_Neutral : Subsystem  VariantControl=Variant3
  Redacted_3288 : Subsystem  VariantControl=Variant2
  Redacted_435 : PMIOPort  Side=Left
  Redacted_1376 : PMIOPort  Port=2  Side=Left
  Redacted_8237 : PMIOPort  Port=3  Side=Left
  Redacted_4941 : PMIOPort  Port=4  Side=Right
  Redacted_729 : PMIOPort  Port=5  Side=Right

== system Electrical_System_2018b_obfs/Redacted_1221/Redacted_7996/Redacted_1/Redacted_4377/Redacted_6082/Redacted_9716 ==
  Redacted_2211 : fl_lib/Electrical/Electrical Elements/Switch  R_closed=afyfvzfsch Ohm  G_open=vrjvijaozw 1/Ohm  Threshold=mknwtzzshw  i_specify=off  i_priority=None  i=ekdwfleukp A  i_nominal_specify=off  i_nominal_unit=A  i_nominal_value=jzjjfeiisz  v_specify=off  v_priority=None  v=phblpacdsh V  v_nominal_specify=off  v_nominal_unit=V  v_nominal_value=bixtyrioal
      settings: SourceProductName=Simscape
  Redacted_2530 : ee_lib/Passive/Thermal/Thermal Resistor  R=eknqnehjdz K/W  T_specify=off  T_priority=None  T=xkbxmmqbok K  T_nominal_specify=off  T_nominal_unit=K  T_nominal_value=uspulwyluj  Q_specify=off  Q_priority=None  Q=rhguguoadf W  Q_nominal_specify=off  Q_nominal_unit=W  Q_nominal_value=scshapasam
      settings: SourceProductName=Simscape Electrical  SourceProductBaseCode=PS  InternalSimscapePortConfiguration="{\"Bottom\":[],\"Left\":[{\"id\":\"A\",\"label\":\"A\",\"type\":\"foundation.thermal.thermal\"}],\"Right\":[{\"id\":\"B\",\"label\":\"B\",\"type\":\"foundation.thermal.thermal\"}],\"Top\":[]}"
  Redacted_2535 : fl_lib/Electrical/Electrical Elements/Switch  R_closed=vipahyjxum Ohm  G_open=dlxajntqoy 1/Ohm  Threshold=twqpdzzoaf  i_specify=off  i_priority=None  i=xisgmotjdl A  i_nominal_specify=off  i_nominal_unit=A  i_nominal_value=hadolbanma  v_specify=off  v_priority=None  v=qlfhrefcfm V  v_nominal_specify=off  v_nominal_unit=V  v_nominal_value=olqxcuwcnl
      settings: SourceProductName=Simscape
  Redacted_5860 : ee_lib/Semiconductors & Converters/Diode  ModelType=yfqphuljkq  Vf=mzcbuksivh V  Ron=hzecvpmxhn Ohm  Goff=tvxqzyuejr S  prmExp=dcqbxdyhji  I12=zqiwcxocbb A  V12=xhqquwuchn V  IS=jximnautsn A  ec=wjykamkomp  I1=pvxecgtjpf A  V1=oldzsjcpiw V  RS=azeneflaop Ohm  Tmeas=xgoovurdtq degC  N_series=ffbptmmmww  N_parallel=pzubandgjz  Rz=nzbxzvjnyf Ohm  BV=jfsodjpvfv V  C_param=xnqrvvpprg  CJ=soexlnhvgu pF  CJ0=cvkocewhza pF  VJ=yygrppicrq V  Mgrad=gytyhuvisu  Vvec=rxofiqevyo V  Cvec=kvpqnhxopf pF  FC=mjsxtxxzuc  Q_param=bbohbnqftg  iRM=nzrtjwpdml A  iF=kbhrbmnbpm A  didt=ptydkofdhp A/us  trr_factor=ejsowqvvzb  trr=mbhiwupcpw ns  Qrr=zrtsqqjyfi s*uA  TT=qevuwyqmgo ns  tau=xolnziyrrw ns  T_param=ljbxpxyrel  IS_T2=iyoqjnnklq A  I1_T2=nbgceqibrt A  V1_T2=gkzwlaxbjv V  Tmeas2=nbfucexxba degC  EG_param=vzpcxvylaa  EG=gwwghaoimg eV  XTI_param=vouzqwssih  XTI=ayunwrccbb  dBVdT=xycjtokfmm V/K  Tdevice=xwhfsoentx degC  i_specify=off  i_priority=None  i=scwomfgbul A  i_nominal_specify=off  i_nominal_unit=A  i_nominal_value=zczgphwnzk  v_specify=off  v_priority=None  v=ycizslduby V  v_nominal_specify=off  v_nominal_unit=V  v_nominal_value=finrjfwbob  i_capacitor_specify=off  i_capacitor_priority=None  i_capacitor=eigdrymvfj A  i_capacitor_nominal_specify=off  i_capacitor_nominal_unit=A  i_capacitor_nominal_value=onrburivct  v_capacitor_specify=off  v_capacitor_priority=None  v_capacitor=vgugbhlxwf V  v_capacitor_nominal_specify=off  v_capacitor_nominal_unit=V  v_capacitor_nominal_value=vlgpvgiuar  power_dissipated_specify=off  power_dissipated_priority=None  power_dissipated=fetinfdjod W  power_dissipated_nominal_specify=off  power_dissipated_nominal_unit=W  power_dissipated_nominal_value=zidttfmnru  thermal_network_parameterization=ebyidfsfgs  Rth=maccbgnykm K/W  Rth_Foster=qrtjgydfwg K/W  thermal_mass_parameterization=ecrfpvdiid  thermal_mass=fhykxyvnrq J/K  thermal_mass_Foster=xqiajsshbg J/K  thermal_time_constant=jmewfaailq s  thermal_time_constant_Foster=iaunggelsj s  thermal_mass_initial_temperatures=eyowrijnjq degC
      settings: SourceProductName=Simscape Electrical  InternalSimscapePortConfiguration="{\"Bottom\":[],\"Left\":[{\"id\":\"p\",\"label\":\"\",\"type\":\"foundation.electrical.electrical\"},{\"id\":\"H\",\"label\":\"H\",\"type\":\"foundation.thermal.thermal\"}],\"Right\":[{\"id\":\"n\",\"label\":\"\",\"type\":\"foundation.electrical.electrical\"}],\"Top\":[]}"
  Redacted_674 : ee_lib/Semiconductors & Converters/Diode  ModelType=wnlytdblho  Vf=sydfdefpdl V  Ron=vdtyquczba Ohm  Goff=wlpgxyumvz S  prmExp=qqfslhfakl  I12=dapzsunzny A  V12=umgrisqttm V  IS=iiuruqhkjg A  ec=qxtumaukto  I1=bemfrijrlo A  V1=ewkugrabqg V  RS=lzmnhodzoo Ohm  Tmeas=tzfyatvwgu degC  N_series=exhrcmoovx  N_parallel=nkjpwtipxm  Rz=qpgvuhphqd Ohm  BV=imeqkbiizq V  C_param=jfyznymhjq  CJ=jrkuonobvh pF  CJ0=qxsplnopwm pF  VJ=wiantwgykb V  Mgrad=uxxbnsjmhs  Vvec=gkwowlpelk V  Cvec=sbymxcpoqv pF  FC=bwazcbkmpz  Q_param=kdshgpaqex  iRM=uffktzxpuq A  iF=pefkqpwhdr A  didt=tiibscarrn A/us  trr_factor=uupbkvcsjn  trr=iirkmlcnco ns  Qrr=mcbhomfcgx s*uA  TT=yhlkukxysz ns  tau=gbtlpwlsum ns  T_param=qqhirjsaof  IS_T2=ussydknlaj A  I1_T2=xeonuwgqet A  V1_T2=saqvtwuqvp V  Tmeas2=nywydxatpl degC  EG_param=cmfbafczlw  EG=hbkkkzznjk eV  XTI_param=gnyhahbixv  XTI=pwmgvjoecr  dBVdT=gveehfslvr V/K  Tdevice=zvkdbgqalk degC  i_specify=off  i_priority=None  i=prekfakgdl A  i_nominal_specify=off  i_nominal_unit=A  i_nominal_value=zusuayujpq  v_specify=off  v_priority=None  v=qpwcvzunkf V  v_nominal_specify=off  v_nominal_unit=V  v_nominal_value=qqnctjlnkc  i_capacitor_specify=off  i_capacitor_priority=None  i_capacitor=mmyvsdgxgm A  i_capacitor_nominal_specify=off  i_capacitor_nominal_unit=A  i_capacitor_nominal_value=gblcdyeldb  v_capacitor_specify=off  v_capacitor_priority=None  v_capacitor=byvhdfymju V  v_capacitor_nominal_specify=off  v_capacitor_nominal_unit=V  v_capacitor_nominal_value=hjxirgzonu  power_dissipated_specify=off  power_dissipated_priority=None  power_dissipated=hksbzjxlmk W  power_dissipated_nominal_specify=off  power_dissipated_nominal_unit=W  power_dissipated_nominal_value=wnwzimuahb  thermal_network_parameterization=vsfmycqswy  Rth=jwzcjrqavw K/W  Rth_Foster=jcpthmykbp K/W  thermal_mass_parameterization=nurvujuzxm  thermal_mass=zmeefhppqv J/K  thermal_mass_Foster=fnpkuytqsg J/K  thermal_time_constant=yslzlhlvpu s  thermal_time_constant_Foster=puzgxzaqxj s  thermal_mass_initial_temperatures=lrnjyzudqy degC
      settings: SourceProductName=Simscape Electrical  InternalSimscapePortConfiguration="{\"Bottom\":[],\"Left\":[{\"id\":\"p\",\"label\":\"\",\"type\":\"foundation.electrical.electrical\"},{\"id\":\"H\",\"label\":\"H\",\"type\":\"foundation.thermal.thermal\"}],\"Right\":[{\"id\":\"n\",\"label\":\"\",\"type\":\"foundation.electrical.electrical\"}],\"Top\":[]}"
  Redacted_8246 : ee_lib/Passive/Thermal/Thermal Resistor  R=pkgfvsjzov K/W  T_specify=off  T_priority=None  T=qxqogaspyo K  T_nominal_specify=off  T_nominal_unit=K  T_nominal_value=mdkgfzcqww  Q_specify=off  Q_priority=None  Q=gomvnbdjkd W  Q_nominal_specify=off  Q_nominal_unit=W  Q_nominal_value=paqpvtpjva
      settings: SourceProductName=Simscape Electrical  SourceProductBaseCode=PS  InternalSimscapePortConfiguration="{\"Bottom\":[],\"Left\":[{\"id\":\"A\",\"label\":\"A\",\"type\":\"foundation.thermal.thermal\"}],\"Right\":[{\"id\":\"B\",\"label\":\"B\",\"type\":\"foundation.thermal.thermal\"}],\"Top\":[]}"
  Redacted_890 : ee_lib/Passive/Thermal/Thermal Resistor  R=djijwylxea K/W  T_specify=off  T_priority=None  T=wauopubvvk K  T_nominal_specify=off  T_nominal_unit=K  T_nominal_value=lrbariemdh  Q_specify=off  Q_priority=None  Q=yuolohvssr W  Q_nominal_specify=off  Q_nominal_unit=W  Q_nominal_value=aqcopqueqm
      settings: SourceProductName=Simscape Electrical  SourceProductBaseCode=PS  InternalSimscapePortConfiguration="{\"Bottom\":[],\"Left\":[{\"id\":\"A\",\"label\":\"A\",\"type\":\"foundation.thermal.thermal\"}],\"Right\":[{\"id\":\"B\",\"label\":\"B\",\"type\":\"foundation.thermal.thermal\"}],\"Top\":[]}"
  Redacted_7205 : PMIOPort  Side=Left
  Redacted_8062 : PMIOPort  Port=2  Side=Left
  Redacted_5929 : PMIOPort  Port=3  Side=Right
  Redacted_7061 : PMIOPort  Port=4  Side=Right
  Redacted_3953 : PMIOPort  Port=5  Side=Left
  Redacted_6306 : PMIOPort  Port=6  Side=Right
  connections:
  Redacted_5860/LConn1 -- Redacted_8062/RConn1
  Redacted_5860/RConn1 -- Redacted_2535/LConn1
  Redacted_674/LConn2 -- Redacted_890/LConn1
  Redacted_5929/RConn1 -- Redacted_2211/RConn2
  Redacted_674/LConn1 -- Redacted_2211/LConn1
  Redacted_7205/RConn1 -- Redacted_674/RConn1
  Redacted_8246/RConn1 -- Redacted_2530/LConn1 -- Redacted_890/RConn1
  Redacted_6306/RConn1 -- Redacted_2535/RConn1 -- Redacted_2211/RConn1
  Redacted_7061/RConn1 -- Redacted_2535/RConn2
  Redacted_2530/RConn1 -- Redacted_3953/RConn1
  Redacted_5860/LConn2 -- Redacted_8246/LConn1
